simulink model "E_1"  (R2020a)
settings: Solver=VariableStepAuto  StartTime=0.0  StopTime=10  RelTol=1e-3
settings Model: Creator=Santiago  LastModifiedBy=Santiago

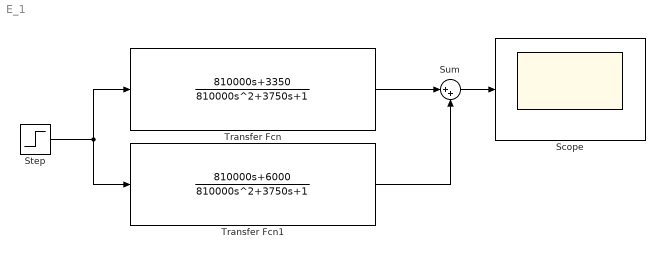
== system E_1 ==
  Scope : Scope
  Step : Step  Time=3  After=20  SampleTime=1
  Sum : Sum  Inputs=|++
  Transfer Fcn : TransferFcn  Numerator=[810000 3350]  Denominator=[810000 3750 1]
  Transfer Fcn1 : TransferFcn  Numerator=[810000 6000]  Denominator=[810000 3750 1]
  wires:
  Step/1 -> Transfer Fcn1/1, Transfer Fcn/1
  Transfer Fcn1/1 -> Sum/2
  Transfer Fcn/1 -> Sum/1
  Sum/1 -> Scope/1
